simulink library "mylib"  (R2018a)
settings: Solver=VariableStepAuto  StartTime=0.0  StopTime=10.0  RelTol=1e-3
settings Model: Creator=toxic  LastModifiedBy=toxic

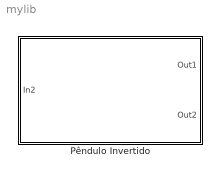
== system mylib ==
  Pêndulo Invertido : Subsystem  mask{m=0.16985, Mc=0.5676, J=0.0032, l=0.478, Beq=5.4, Bp=0.0024, g=9.81, ang_init=0, pos_init=0, vel_init=0, vel_ang_init=0}
      mask prompts: m "Massa pêndulo (kg)"; Mc "Massa do carro (kg)"; J "Momento de inércia do pêndulo"; l "Tamanho da haste (m)"; Beq "Coeficiente viscoso de amortecimento do carro"; Bp "Coeficiente viscoso de amortecimento rotacional do pêndulo"; g "Aceleração da gravidade"; ang_init "Ângulo Inicial (rad)"; pos_init "Posição Inicial (m)"; vel_init "Velocidade linear inicial (m/s)"; vel_ang_init "Velocidade angular inicial (rad/s)"
      mask DialogControl DescGroupVar Prompt: Pêndulo Invertido
      mask DialogControl ParameterGroupVar Prompt: Parâmetros do sistema
      mask DialogControl Container3 Prompt: Condições Iniciais

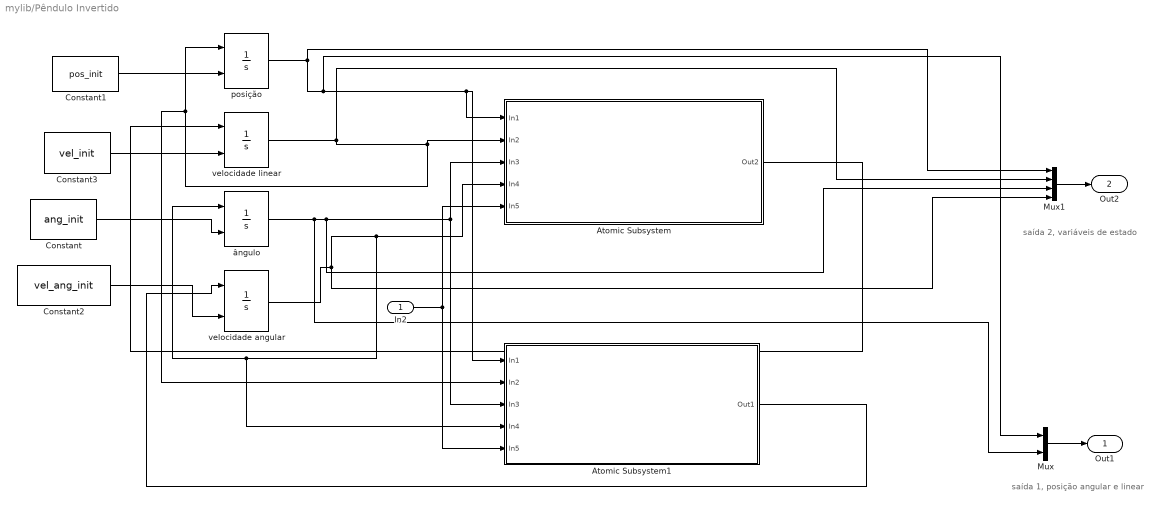
== system mylib/Pêndulo Invertido ==
  note: saída 2, variáveis de estado
  note: saída 1, posição angular e linear
  In2 : Inport
  Atomic Subsystem : Subsystem  TreatAsAtomicUnit=on
  Atomic Subsystem1 : Subsystem  TreatAsAtomicUnit=on
  Constant : Constant  Value=ang_init
  Constant1 : Constant  Value=pos_init
  Constant2 : Constant  Value=vel_ang_init
  Constant3 : Constant  Value=vel_init
  Mux : Mux  Inputs=2
  Mux1 : Mux
  "posição " : Integrator  InitialConditionSource=external
  velocidade angular : Integrator  InitialConditionSource=external
  velocidade linear : Integrator  InitialConditionSource=external
  ângulo : Integrator  InitialConditionSource=external  InitialCondition=0.52
  Out1 : Outport
  Out2 : Outport  Port=2
  wires:
  Atomic Subsystem/1(Out2) -> velocidade linear/1
  "posição "/1 -> Mux/1, Atomic Subsystem1/1(In1), Atomic Subsystem/1(In1), Mux1/1
  In2/1 -> Atomic Subsystem/5(In5), Atomic Subsystem1/5(In5)
  Atomic Subsystem1/1(Out1) -> velocidade angular/1
  ângulo/1 -> Mux1/3, Atomic Subsystem/3(In3), Atomic Subsystem1/3(In3), Mux/2
  velocidade linear/1 -> Atomic Subsystem/2(In2), "posição "/1, Atomic Subsystem1/2(In2), Mux1/2
  velocidade angular/1 -> ângulo/1, Atomic Subsystem1/4(In4), Atomic Subsystem/4(In4), Mux1/4
  Mux/1 -> Out1/1
  Mux1/1 -> Out2/1
  Constant/1 -> ângulo/2
  Constant1/1 -> "posição "/2
  Constant2/1 -> velocidade angular/2
  Constant3/1 -> velocidade linear/2

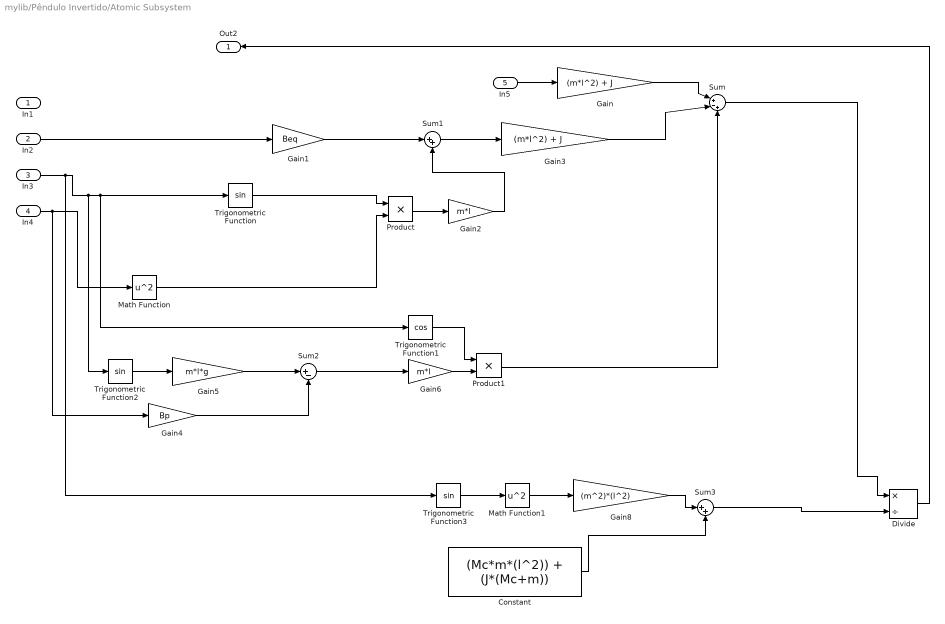
== system mylib/Pêndulo Invertido/Atomic Subsystem ==
  In1 : Inport
  In2 : Inport  Port=2
  In3 : Inport  Port=3
  In4 : Inport  Port=4
  In5 : Inport  Port=5
  Constant : Constant  Value=(Mc*m*(l^2)) + (J*(Mc+m))
  Divide : Product  Inputs=*/
  Gain : Gain  Gain=(m*l^2) + J
  Gain1 : Gain  Gain=Beq
  Gain2 : Gain  Gain=m*l
  Gain3 : Gain  Gain=(m*l^2) + J
  Gain4 : Gain  Gain=Bp
  Gain5 : Gain  Gain=m*l*g
  Gain6 : Gain  Gain=m*l
  Gain8 : Gain  Gain=(m^2)*(l^2)
  Math Function : Math  Operator=square  SaturateOnIntegerOverflow=on
  Math Function1 : Math  Operator=square  SaturateOnIntegerOverflow=on
  Product : Product
  Product1 : Product
  Sum : Sum  Inputs=|+-+
  Sum1 : Sum  Inputs=|++
  Sum2 : Sum  Inputs=|+-
  Sum3 : Sum  Inputs=|++
  Trigonometric Function : Trigonometry
  Trigonometric Function1 : Trigonometry  Operator=cos
  Trigonometric Function2 : Trigonometry
  Trigonometric Function3 : Trigonometry
  Out2 : Outport
  wires:
  Gain4/1 -> Sum2/2
  Gain1/1 -> Sum1/1
  Gain6/1 -> Product1/2
  Sum2/1 -> Gain6/1
  Trigonometric Function/1 -> Product/1
  Sum1/1 -> Gain3/1
  Math Function/1 -> Product/2
  Sum3/1 -> Divide/2
  Gain8/1 -> Sum3/1
  Constant/1 -> Sum3/2
  Product/1 -> Gain2/1
  Product1/1 -> Sum/3
  Gain/1 -> Sum/1
  Gain3/1 -> Sum/2
  Gain2/1 -> Sum1/2
  Sum/1 -> Divide/1
  Trigonometric Function1/1 -> Product1/1
  Math Function1/1 -> Gain8/1
  Gain5/1 -> Sum2/1
  In2/1 -> Gain1/1
  In4/1 -> Gain4/1, Math Function/1
  In3/1 -> Trigonometric Function3/1, Trigonometric Function2/1, Trigonometric Function1/1, Trigonometric Function/1
  Trigonometric Function2/1 -> Gain5/1
  Trigonometric Function3/1 -> Math Function1/1
  Divide/1 -> Out2/1
  In5/1 -> Gain/1

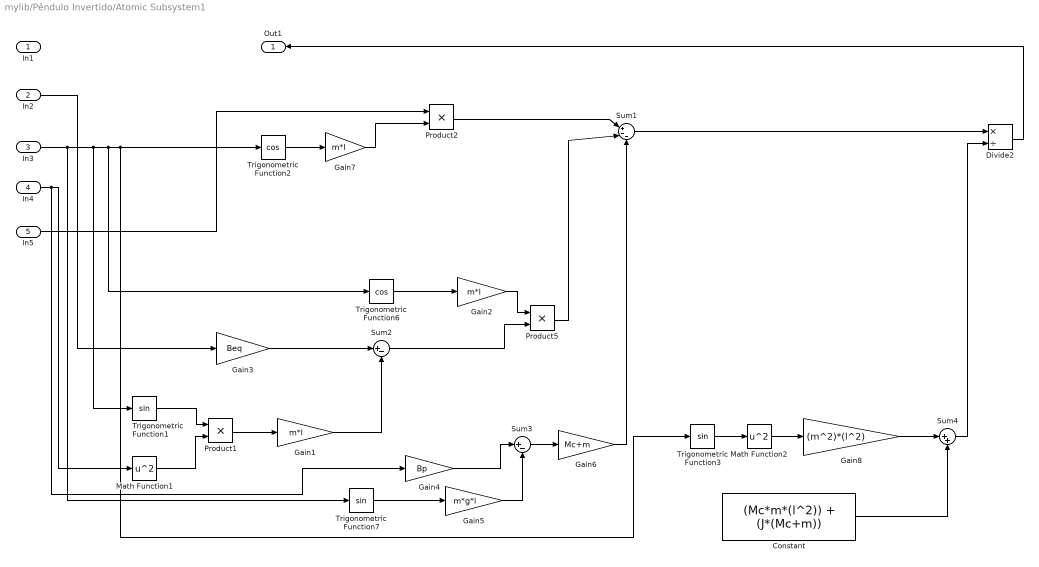
== system mylib/Pêndulo Invertido/Atomic Subsystem1 ==
  In1 : Inport
  In2 : Inport  Port=2
  In3 : Inport  Port=3
  In4 : Inport  Port=4
  In5 : Inport  Port=5
  Constant : Constant  Value=(Mc*m*(l^2)) + (J*(Mc+m))
  Divide2 : Product  Inputs=*/
  Gain1 : Gain  Gain=m*l
  Gain2 : Gain  Gain=m*l
  Gain3 : Gain  Gain=Beq
  Gain4 : Gain  Gain=Bp
  Gain5 : Gain  Gain=m*g*l
  Gain6 : Gain  Gain=Mc+m
  Gain7 : Gain  Gain=m*l
  Gain8 : Gain  Gain=(m^2)*(l^2)
  Math Function1 : Math  Operator=square  SaturateOnIntegerOverflow=on
  Math Function2 : Math  Operator=square  SaturateOnIntegerOverflow=on
  Product1 : Product
  Product2 : Product
  Product5 : Product
  Sum1 : Sum  Inputs=|+--
  Sum2 : Sum  Inputs=|+-
  Sum3 : Sum  Inputs=|+-
  Sum4 : Sum  Inputs=|++
  Trigonometric Function1 : Trigonometry
  Trigonometric Function2 : Trigonometry  Operator=cos
  Trigonometric Function3 : Trigonometry
  Trigonometric Function6 : Trigonometry  Operator=cos
  Trigonometric Function7 : Trigonometry
  Out1 : Outport
  wires:
  Trigonometric Function2/1 -> Gain7/1
  Gain7/1 -> Product2/2
  In5/1 -> Product2/1
  In3/1 -> Trigonometric Function7/1, Trigonometric Function1/1, Trigonometric Function6/1, Trigonometric Function3/1, Trigonometric Function2/1
  Product2/1 -> Sum1/1
  Math Function1/1 -> Product1/2
  Gain3/1 -> Sum2/1
  Trigonometric Function1/1 -> Product1/1
  Sum2/1 -> Product5/2
  Product1/1 -> Gain1/1
  Gain2/1 -> Product5/1
  Trigonometric Function6/1 -> Gain2/1
  Gain1/1 -> Sum2/2
  In2/1 -> Gain3/1
  In4/1 -> Gain4/1, Math Function1/1
  Product5/1 -> Sum1/2
  Sum3/1 -> Gain6/1
  Gain5/1 -> Sum3/2
  Trigonometric Function7/1 -> Gain5/1
  Gain4/1 -> Sum3/1
  Gain6/1 -> Sum1/3
  Sum1/1 -> Divide2/1
  Trigonometric Function3/1 -> Math Function2/1
  Gain8/1 -> Sum4/1
  Constant/1 -> Sum4/2
  Math Function2/1 -> Gain8/1
  Sum4/1 -> Divide2/2
  Divide2/1 -> Out1/1
